simulink model "Simulink_mod_index_AM_Mod_Demod"  (R2021a)
settings: Solver=VariableStepAuto  StartTime=0.0  StopTime=10.0  RelTol=1e-3
libraries: dspfdesign x1
settings Model: Creator=visha  LastModifiedBy=visha

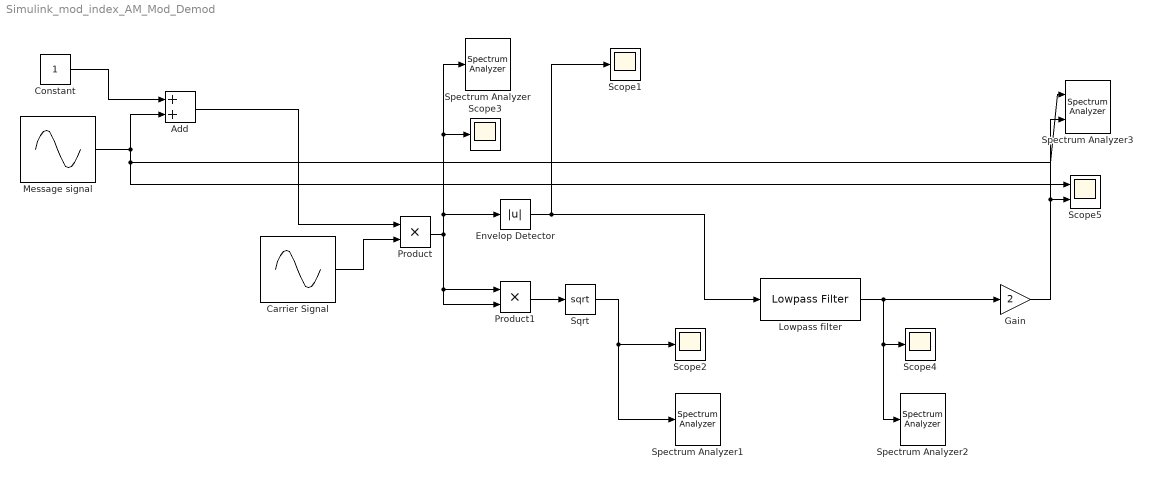
== system Simulink_mod_index_AM_Mod_Demod ==
  Add : Sum
  Carrier Signal : Sin  Frequency=1000*2*pi  Phase=pi/2  SampleTime=1/2^14
  Constant : Constant
  Envelop Detector : Abs
  Gain : Gain  Gain=2
  Lowpass filter : dspfdesign/Lowpass Filter  FilterType=FIR  DesignForMinimumOrder=on  FilterOrder=50  PassbandFrequency=0.1e3  StopbandFrequency=1e3  PassbandRipple=0.1  StopbandAttenuation=80  InheritSampleRate=off  SampleRate=44100  SimulateUsing=Interpreted execution  roundingMode=Floor  coeffsDataTypeStr=fixdt(1,16)
  Message signal : Sin  Frequency=100*2*pi  SampleTime=1/2^14
  Product : Product
  Product1 : Product
  Scope{1..4} (4 alike) : Scope
  Scope5 : Scope  NumInputPorts=2
  Spectrum Analyzer : SpectrumAnalyzer
  Spectrum Analyzer1 : SpectrumAnalyzer
  Spectrum Analyzer2 : SpectrumAnalyzer
  Spectrum Analyzer3 : SpectrumAnalyzer  NumInputPorts=2
  Sqrt : Sqrt  SaturateOnIntegerOverflow=on
  wires:
  Lowpass filter/1 -> Gain/1, Spectrum Analyzer2/1, Scope4/1
  Gain/1 -> Spectrum Analyzer3/2, Scope5/2
  Product/1 -> Envelop Detector/1, Spectrum Analyzer/1, Scope3/1, Product1/2, Product1/1
  Carrier Signal/1 -> Product/2
  Constant/1 -> Add/1
  Message signal/1 -> Spectrum Analyzer3/1, Scope5/1, Add/2
  Add/1 -> Product/1
  Envelop Detector/1 -> Scope1/1, Lowpass filter/1
  Sqrt/1 -> Spectrum Analyzer1/1, Scope2/1
  Product1/1 -> Sqrt/1
